simulink model "RollControl_OpenLoop"  (R2024b)
settings: Solver=VariableStepAuto  StartTime=0.0  StopTime=10  RelTol=1e-3
settings Model: Creator=Arghya  LastModifiedBy=Arghya

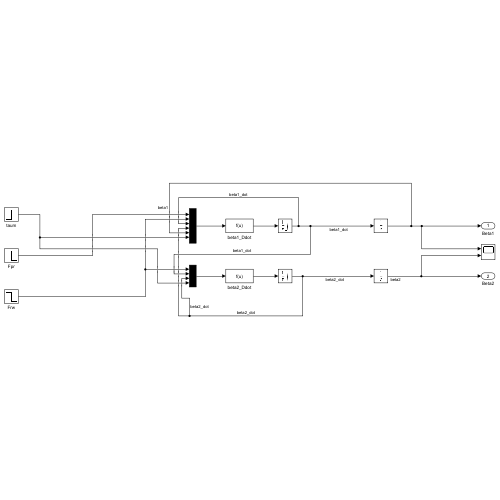
[thumbnail: Simulink's stored preview of the top-level diagram]
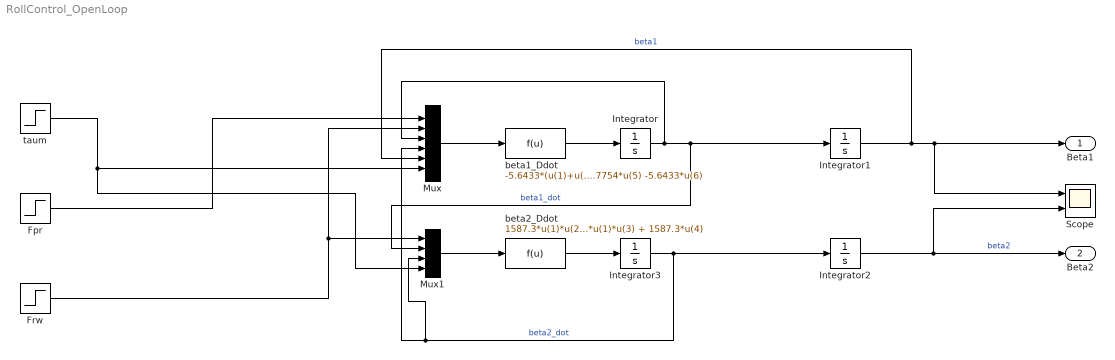
== system RollControl_OpenLoop ==
  Fpr : Step  Before=1  After=0  SampleTime=0.3
  Frw : Step  Before=1  After=0  SampleTime=0.3
  Integrator : Integrator  LimitOutput=on  UpperSaturationLimit=pi/2  LowerSaturationLimit=-pi/2  ContinuousStateAttributes="\"beta1_dot\""
  Integrator1 : Integrator  UpperSaturationLimit=pi/2  LowerSaturationLimit=-pi/2  ContinuousStateAttributes="\"beta1\""
  Integrator2 : Integrator  UpperSaturationLimit=2*pi  LowerSaturationLimit=0  ContinuousStateAttributes="\"beta2\""
  Integrator3 : Integrator  LimitOutput=on  UpperSaturationLimit=2*pi  LowerSaturationLimit=0  ContinuousStateAttributes="\"beta2_dot\""
  Mux : Mux  Inputs=6
  Mux1 : Mux
  Scope : Scope  NumInputPorts=2
  beta1_Ddot : Fcn  Expr=-5.6433*(u(1)+u(2))*u(3) + 5.6433*u(4) - 94.7754*u(5) -5.6433*u(6)
  beta2_Ddot : Fcn  Expr=1587.3*u(1)*u(2) - 1587.3*u(1)*u(3) + 1587.3*u(4)
  taum : Step  SampleTime=0
  Beta1 : Outport
  Beta2 : Outport  Port=2
  wires:
  beta1_Ddot/1 -> Integrator/1
  Integrator/1 -> Mux/3, Mux1/2, Integrator1/1  "beta1_dot"
  beta2_Ddot/1 -> Integrator3/1
  Integrator3/1 -> Mux1/3, Mux/4, Integrator2/1  "beta2_dot"
  Integrator1/1 -> Mux/5, Scope/1, Beta1/1  "beta1"
  Fpr/1 -> Mux/1
  Frw/1 -> Mux1/1, Mux/2
  Mux/1 -> beta1_Ddot/1
  Mux1/1 -> beta2_Ddot/1
  Integrator2/1 -> Scope/2, Beta2/1  "beta2"
  taum/1 -> Mux1/4, Mux/6
